simulink model "model_without_discrete"  (R2022a)
settings: Solver=VariableStepAuto  StartTime=0.0  StopTime=10.0  RelTol=1e-6
values from neighbouring files (symbols this model uses):
  K_oc = 1.2    [task1.m]
  K_oy = 9.8    [config.m]
settings Model: Creator=Vvlad  LastModifiedBy=Vvlad

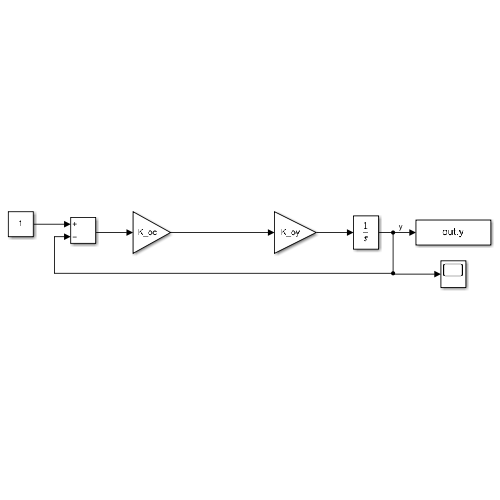
[thumbnail: Simulink's stored preview of the top-level diagram]
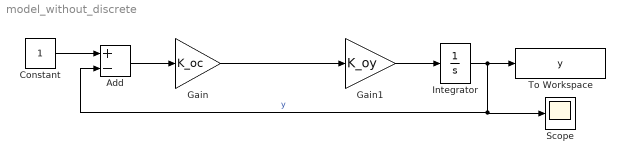
== system model_without_discrete ==
  Add : Sum  Inputs=+-
  Constant : Constant
  Gain : Gain  Gain=K_oc
  Gain1 : Gain  Gain=K_oy
  Integrator : Integrator
  Scope : Scope
  To Workspace : ToWorkspace  VariableName=y  SampleTime=-1
  wires:
  Add/1 -> Gain/1
  Gain1/1 -> Integrator/1
  Integrator/1 -> To Workspace/1, Scope/1, Add/2  "y"
  Gain/1 -> Gain1/1
  Constant/1 -> Add/1
